simulink model "serialTest"  (R2020a)
settings: Solver=FixedStepAuto  StartTime=0.0  StopTime=10.0  FixedStep=1e-3  RelTol=1e-3  EnableMultiTasking=on
libraries: frdmk64flib x4
settings Model: ExtModeTrigDuration=5  Creator=Liam  LastModifiedBy=Liam
settings OptimizationCC: EnhancedBackFolding=on  PassReuseOutputArgsAs=Individual arguments  ZeroExternalMemoryAtStartup=off  ZeroInternalMemoryAtStartup=off  MaxStackSize=64  OptimizeBlockOrder=speed  DifferentSizesBufferReuse=on  OptimizationCustomize=off  EfficientTunableParamExpr=on
settings DebuggingCC: ParameterTunabilityLossMsg=error
settings HardwareCC: ProdBitPerPointer=32  ProdBitPerSizeT=32  ProdBitPerPtrDiffT=32  ProdLargestAtomicInteger=Long  ProdLargestAtomicFloat=Double  ProdWordSize=32  ProdHWDeviceType=ARM Compatible->ARM Cortex
settings SFSimCC: MATLABDynamicMemAlloc=off
settings RTWCC: SystemTargetFile=ert.tlc  HardwareBoard=NXP FRDM-K64F  TemplateMakefile=ert_default_tmf  Toolchain=GNU Tools for ARM Embedded Processors
settings CodeAppCC: ForceParamTrailComments=on  IgnoreCustomStorageClasses=off  OperatorAnnotations=on  SimulinkDataObjDesc=on  SFDataObjDesc=on  InsertBlockDesc=on

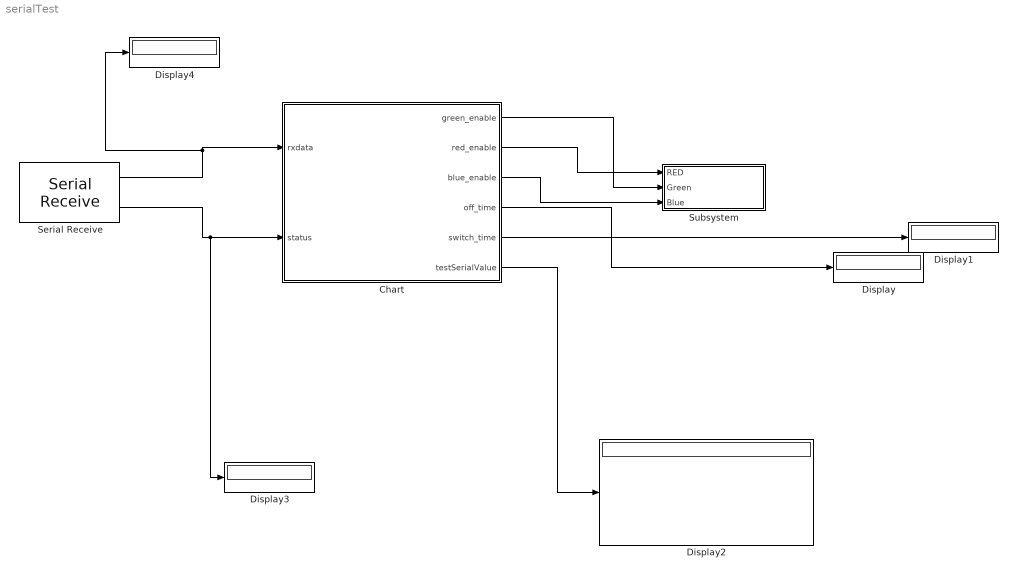
== system serialTest ==
  Chart : Stateflow chart  TreatAsAtomicUnit=on
  Display{,1..4} (5 alike) : Display
  Serial Receive : frdmk64flib/Serial Receive  SCIModule=0  Baudrate=uint32(9600)  Parity=None  StopBits=1  HardwareFlowControl=None  ByteOrder=LittleEndian  DataType=uint8  DataLength=10  BlockingMode=off  OutputStatus=on  SampleTime=0.1
  Subsystem : Subsystem
  wires:
  Serial Receive/1 -> Display4/1, Chart/1(rxdata)
  Serial Receive/2 -> Display3/1, Chart/2(status)
  Chart/1(green_enable) -> Subsystem/2(Green)
  Chart/2(red_enable) -> Subsystem/1(RED)
  Chart/3(blue_enable) -> Subsystem/3(Blue)
  Chart/4(off_time) -> Display/1
  Chart/5(switch_time) -> Display1/1
  Chart/6(testSerialValue) -> Display2/1

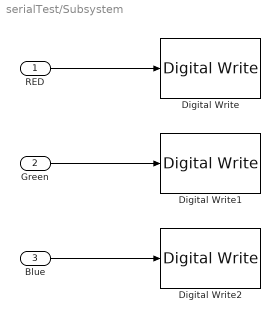
== system serialTest/Subsystem ==
  RED : Inport
  Green : Inport  Port=2
  Blue : Inport  Port=3
  Digital Write : frdmk64flib/Digital Write  Whichpin=RED_LED
  Digital Write1 : frdmk64flib/Digital Write  Whichpin=GREEN_LED
  Digital Write2 : frdmk64flib/Digital Write  Whichpin=BLUE_LED
  wires:
  RED/1 -> Digital Write/1
  Green/1 -> Digital Write1/1
  Blue/1 -> Digital Write2/1

== stateflow chart serialTest/Chart ==
  state SET_PARAM
    entry:
    red_enable =rxdata(3);
    green_enable=rxdata(4);
    blue_enable=rxdata(5);
    off_time= typecast(rxdata(6:9),'single');
    switch_time= typecast(rxdata(10:11),'uint16')
    testSerialValue=rxdata(3);
  state INITIAL
    entry:
    red_enable=0;
    green_enable=0;
    blue_enable=0;
    off_time=0.5; %in seconds
    switch_time=200% in milliseconds
  state STANDBY
    %wait
  SET_PARAM -> STANDBY
  (default) -> INITIAL
  (junction 6) -> STANDBY [order 2]
  (junction 9) -> SET_PARAM : [rxdata(2)==hex2dec('55')]{green_enable=1}
  INITIAL -> STANDBY
  STANDBY -> (junction 6) : [status==0]{blue_enable=1}
  (junction 6) -> (junction 9) [order 1] : [rxdata(1)==hex2dec('16')]{red_enable=1}
  data: rxdata input uint8; status input uint8; green_enable output uint8; red_enable output uint8; blue_enable output uint8; off_time output single; switch_time output uint16; testSerialValue output
